simulink model "decoder_wt_en"  (R2015a)
settings: Solver=ode45  StartTime=0.0  StopTime=10.0  RelTol=1e-3
settings Model: Creator=Shravankumar  LastModifiedBy=Shravankumar

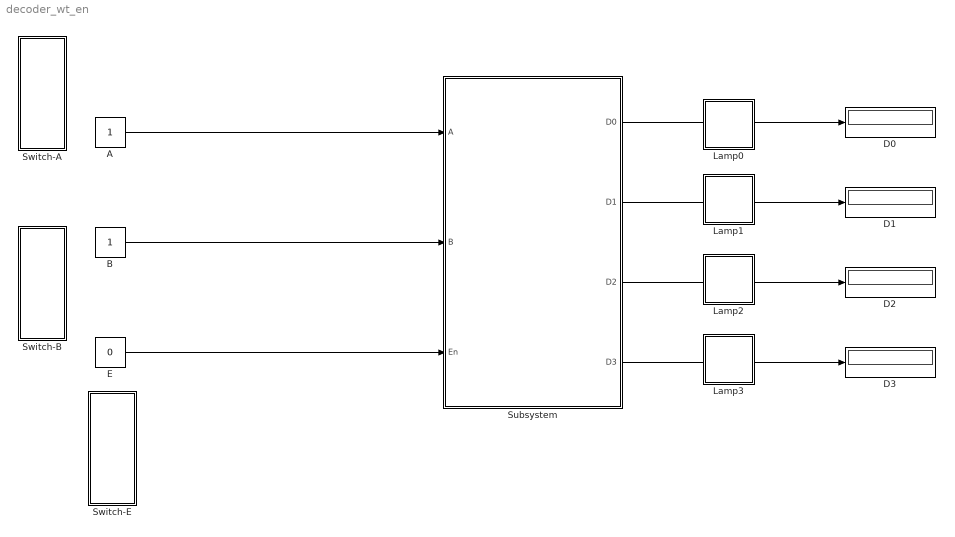
== system decoder_wt_en ==
  A : Constant  OutDataTypeStr=boolean
  B : Constant  OutDataTypeStr=boolean
  D{0..3} (4 alike) : Display
  E : Constant  Value=0  OutDataTypeStr=boolean
  Lamp0 : Subsystem  DialogController=hmiCreateDDGDialog  IsWebBlock=on  mask(MathWorksWebBlock){webBlockId=c9c5711f-9a8e-4087-9d12-66d50f0d01f6, webBlockType=lamp, ShowInLibBrowser=on, ShowInitialText=on, HMISrcModelName=decoder_wt_en}
      mask prompts: webBlockType "WebBlock Type"; HMISrcModelName "Source Model"
      mask Help: helpview([docroot '/mapfiles/simulink.map'], 'hmi_lamp')
      mask Display:
      | if strcmp(get_param(bdroot(gcb),'BlockDiagramType'), 'library')
      |     image([(matlabroot) '/toolbox/simulink/hmi/icons/Lamp.png']);
      | end
  Lamp1 : Subsystem  DialogController=hmiCreateDDGDialog  IsWebBlock=on  mask(MathWorksWebBlock){webBlockId=ca3581ac-bc31-4d4e-b816-a2fccbb3d195, webBlockType=lamp, ShowInLibBrowser=on, ShowInitialText=on, HMISrcModelName=decoder_wt_en}
      mask prompts: webBlockType "WebBlock Type"; HMISrcModelName "Source Model"
      mask Help: helpview([docroot '/mapfiles/simulink.map'], 'hmi_lamp')
      mask Display:
      | if strcmp(get_param(bdroot(gcb),'BlockDiagramType'), 'library')
      |     image([(matlabroot) '/toolbox/simulink/hmi/icons/Lamp.png']);
      | end
  Lamp2 : Subsystem  DialogController=hmiCreateDDGDialog  IsWebBlock=on  mask(MathWorksWebBlock){webBlockId=ce22a557-c41f-44d1-ab6a-242c73e8929c, webBlockType=lamp, ShowInLibBrowser=on, ShowInitialText=on, HMISrcModelName=decoder_wt_en}
      mask prompts: webBlockType "WebBlock Type"; HMISrcModelName "Source Model"
      mask Help: helpview([docroot '/mapfiles/simulink.map'], 'hmi_lamp')
      mask Display:
      | if strcmp(get_param(bdroot(gcb),'BlockDiagramType'), 'library')
      |     image([(matlabroot) '/toolbox/simulink/hmi/icons/Lamp.png']);
      | end
  Lamp3 : Subsystem  DialogController=hmiCreateDDGDialog  IsWebBlock=on  mask(MathWorksWebBlock){webBlockId=7062e4dd-d925-4c8e-8ace-d3c153a711f3, webBlockType=lamp, ShowInLibBrowser=on, ShowInitialText=on, HMISrcModelName=decoder_wt_en}
      mask prompts: webBlockType "WebBlock Type"; HMISrcModelName "Source Model"
      mask Help: helpview([docroot '/mapfiles/simulink.map'], 'hmi_lamp')
      mask Display:
      | if strcmp(get_param(bdroot(gcb),'BlockDiagramType'), 'library')
      |     image([(matlabroot) '/toolbox/simulink/hmi/icons/Lamp.png']);
      | end
  Subsystem : Subsystem
  Switch-A : Subsystem  DialogController=hmiCreateDDGDialog  IsWebBlock=on  mask(MathWorksWebBlock){webBlockId=334e63c9-565e-4641-af15-e28ca346a077, webBlockType=rockerswitch, ShowInLibBrowser=on, ShowInitialText=on, HMISrcModelName=decoder_wt_en}
      mask prompts: webBlockId "WebBlock Id"; webBlockType "WebBlock Type"; HMISrcModelName "Source Model"
      mask Help: helpview([docroot '/mapfiles/simulink.map'], 'hmi_rocker_switch')
      mask Display:
      | if strcmp(get_param(bdroot(gcb),'BlockDiagramType'), 'library')
      |     image([(matlabroot) '/toolbox/simulink/hmi/icons/RockerSwitch.png']);
      | end
  Switch-B : Subsystem  DialogController=hmiCreateDDGDialog  IsWebBlock=on  mask(MathWorksWebBlock){webBlockId=3a6149c4-e0b5-4918-a6dd-4afedaa38971, webBlockType=rockerswitch, ShowInLibBrowser=on, ShowInitialText=on, HMISrcModelName=decoder_wt_en}
      mask prompts: webBlockId "WebBlock Id"; webBlockType "WebBlock Type"; HMISrcModelName "Source Model"
      mask Help: helpview([docroot '/mapfiles/simulink.map'], 'hmi_rocker_switch')
      mask Display:
      | if strcmp(get_param(bdroot(gcb),'BlockDiagramType'), 'library')
      |     image([(matlabroot) '/toolbox/simulink/hmi/icons/RockerSwitch.png']);
      | end
  Switch-E : Subsystem  DialogController=hmiCreateDDGDialog  IsWebBlock=on  mask(MathWorksWebBlock){webBlockId=24bb3259-1032-43ad-8ebd-0d156cb3369e, webBlockType=rockerswitch, ShowInLibBrowser=on, ShowInitialText=on, HMISrcModelName=decoder_wt_en}
      mask prompts: webBlockId "WebBlock Id"; webBlockType "WebBlock Type"; HMISrcModelName "Source Model"
      mask Help: helpview([docroot '/mapfiles/simulink.map'], 'hmi_rocker_switch')
      mask Display:
      | if strcmp(get_param(bdroot(gcb),'BlockDiagramType'), 'library')
      |     image([(matlabroot) '/toolbox/simulink/hmi/icons/RockerSwitch.png']);
      | end
  wires:
  E/1 -> Subsystem/3(En)
  A/1 -> Subsystem/1(A)
  B/1 -> Subsystem/2(B)
  Subsystem/1(D0) -> D0/1
  Subsystem/2(D1) -> D1/1
  Subsystem/3(D2) -> D2/1
  Subsystem/4(D3) -> D3/1

== system decoder_wt_en/Lamp0 ==

== system decoder_wt_en/Lamp1 ==

== system decoder_wt_en/Lamp2 ==

== system decoder_wt_en/Lamp3 ==

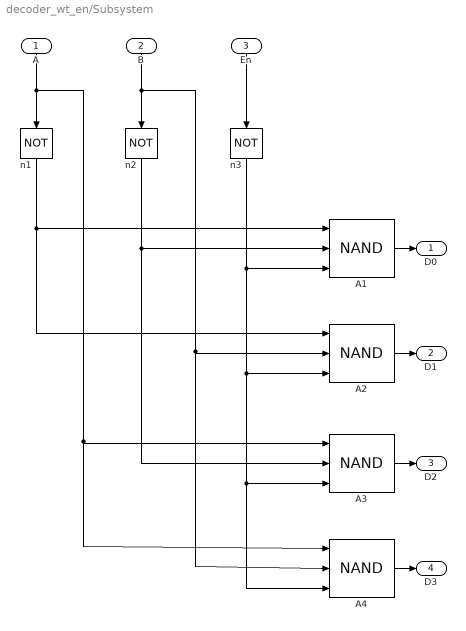
== system decoder_wt_en/Subsystem ==
  A : Inport
  B : Inport  Port=2
  En : Inport  Port=3
  A{1..4} (4 alike) : Logic  Operator=NAND  Inputs=3  IconShape=distinctive  AllPortsSameDT=off  OutDataTypeStr=boolean
  n1 : Logic  Operator=NOT  IconShape=distinctive  AllPortsSameDT=off  OutDataTypeStr=boolean
  n2 : Logic  Operator=NOT  IconShape=distinctive  AllPortsSameDT=off  OutDataTypeStr=boolean
  n3 : Logic  Operator=NOT  IconShape=distinctive  AllPortsSameDT=off  OutDataTypeStr=boolean
  D0 : Outport
  D1 : Outport  Port=2
  D2 : Outport  Port=3
  D3 : Outport  Port=4
  wires:
  En/1 -> n3/1
  B/1 -> A4/2, A2/2, n2/1
  n1/1 -> A2/1, A1/1
  A2/1 -> D1/1
  n2/1 -> A1/2, A3/2
  A/1 -> A4/1, A3/1, n1/1
  A1/1 -> D0/1
  A4/1 -> D3/1
  n3/1 -> A1/3, A2/3, A3/3, A4/3
  A3/1 -> D2/1

== system decoder_wt_en/Switch-A ==

== system decoder_wt_en/Switch-B ==

== system decoder_wt_en/Switch-E ==
